simulink model "trigger"  (R2014a)
settings: Solver=ode45  StartTime=0.0  StopTime=10.0  RelTol=1e-3
undefined symbols (not defined in the file or in its folder): DCT_Param
settings Model: Creator=wnursilo  LastModifiedBy=wnursilo

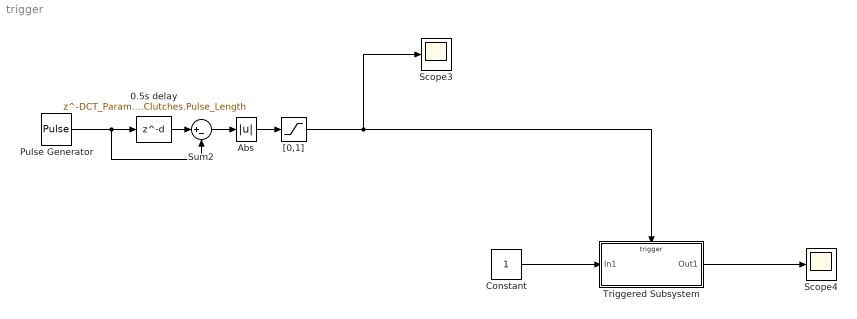
== system trigger ==
  0.5s delay : Delay  DelayLength=DCT_Param.Dog_Clutches.Pulse_Length  SampleTime=0.01
  Abs : Abs  SaturateOnIntegerOverflow=on
  Constant : Constant
  Pulse Generator : DiscretePulseGenerator  PulseType=Time based  PulseWidth=50
  Scope3 : Scope
      settings: SaveName=ScopeData3
  Scope4 : Scope
  Sum2 : Sum  Inputs=|+-  SaturateOnIntegerOverflow=on  InputSameDT=on  OutDataTypeStr=Inherit: Same as first input
  Triggered Subsystem : Subsystem  TreatAsAtomicUnit=on
  "[0,1]" : Saturate  UpperLimit=1  LowerLimit=0
  wires:
  0.5s delay/1 -> Sum2/1
  Sum2/1 -> Abs/1
  Abs/1 -> "[0,1]"/1
  "[0,1]"/1 -> Triggered Subsystem/Trigger, Scope3/1
  Pulse Generator/1 -> Sum2/2, 0.5s delay/1
  Constant/1 -> Triggered Subsystem/1(In1)
  Triggered Subsystem/1(Out1) -> Scope4/1

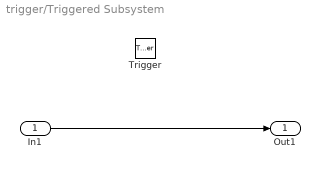
== system trigger/Triggered Subsystem ==
  In1 : Inport
  Trigger : TriggerPort
  Out1 : Outport
  wires:
  In1/1 -> Out1/1
